simulink model "flyback_DT_working(2)"  (R2022b)
settings: Solver=FixedStepDiscrete  StartTime=0.0  StopTime=100e-3  RelTol=1e-3
undefined symbols (not defined in the file): DiscIntNeverNeededParam
libraries: cstblocks x4, simulink x1
Description:
  | Symmetric FIR Filter
  | This example shows how to use HDL Coder(TM) to check, generate,
  | and verify HDL for a fixed-point symmetric FIR filter.
settings Model: DataTypeOverride=Off  Creator=The MathWorks, Inc.  LastModifiedBy=justu
settings SolverCC: AlgebraicLoopSolver=TrustRegion  AutoInsertRateTranBlk=on
settings DataIOCC: LimitDataPoints=on  SaveFormat=Array  SaveOutput=off  SignalLogging=off  SaveTime=off  ReturnWorkspaceOutputs=off  SignalLoggingName=logsOut
settings OptimizationCC: BlockReduction=off  BooleanDataType=off  ConditionallyExecuteInputs=off  DefaultParameterBehavior=Inlined  InheritOutputTypeSmallerThanSingle=on  InlineInvariantSignals=on  ExpressionDepthLimit=2147483647  InitFltsAndDblsToZero=on  LifeSpan=inf  BufferReusableBoundary=off
settings DebuggingCC: AlgebraicLoopMsg=error  SaveWithParameterizedLinksMsg=none  UnderspecifiedInitializationDetection=Classic  MergeDetectMultiDrivingBlocksExec=none  CheckExecutionContextPreStartOutputMsg=on  SignalResolutionControl=TryResolveAllWithWarning  MultiTaskDSMMsg=warning  MultiTaskCondExecSysMsg=none  SingleTaskRateTransMsg=error  IntegerOverflowMsg=none  ParameterPrecisionLossMsg=none  FcnCallInpInsideContextMsg=warning  UnconnectedInputMsg=warning  UnconnectedOutputMsg=warning  UnconnectedLineMsg=warning  BusObjectLabelMismatch=none  StateNameClashWarn=warning  SFUnexpectedBacktrackingDiag=warning  SFNoUnconditionalDefaultTransitionDiag=warning  SFExecutionAtInitializationDiag=none  SFMachineParentedDataDiag=warning  IntegerSaturationMsg=none  ArithmeticOperatorsInVariantConditions=warning
settings HardwareCC: ProdBitPerPointer=32  ProdBitPerSizeT=32  ProdBitPerPtrDiffT=32  ProdLargestAtomicFloat=None  ProdIntDivRoundTo=Undefined  ProdEndianess=Unspecified  ProdWordSize=32  ProdHWDeviceType=ASIC/FPGA  TargetUnknown=on  ProdEqTarget=off
settings ModelReferenceCC: EnableRefExpFcnMdlSchedulingChecks=on  PropagateSignalLabelsOutOfModel=off
settings SFSimCC: SimUseLocalCustomCode=off  CustomCodeUndefinedFunction=UseInterfaceOnly
settings RTWCC: RTWUseLocalCustomCode=off  DLArmComputeVersion=19.05
settings CodeAppCC: StateflowObjectComments=on
settings GRTTargetCC: TargetFcnLib=ansi_tfl_tmw.mat  TargetLangStandard=C89/C90 (ANSI)  CombineOutputUpdateFcns=off  GRTInterface=on
settings ConfigComp: CovMetricSettings=dw  CovSaveCumulativeToWorkspaceVar=on  CovSaveSingleToWorkspaceVar=on  CovExternalEMLEnable=off

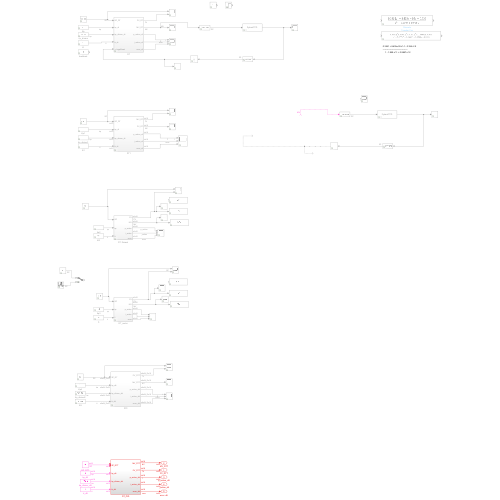
[thumbnail: Simulink's stored preview of the top-level diagram]
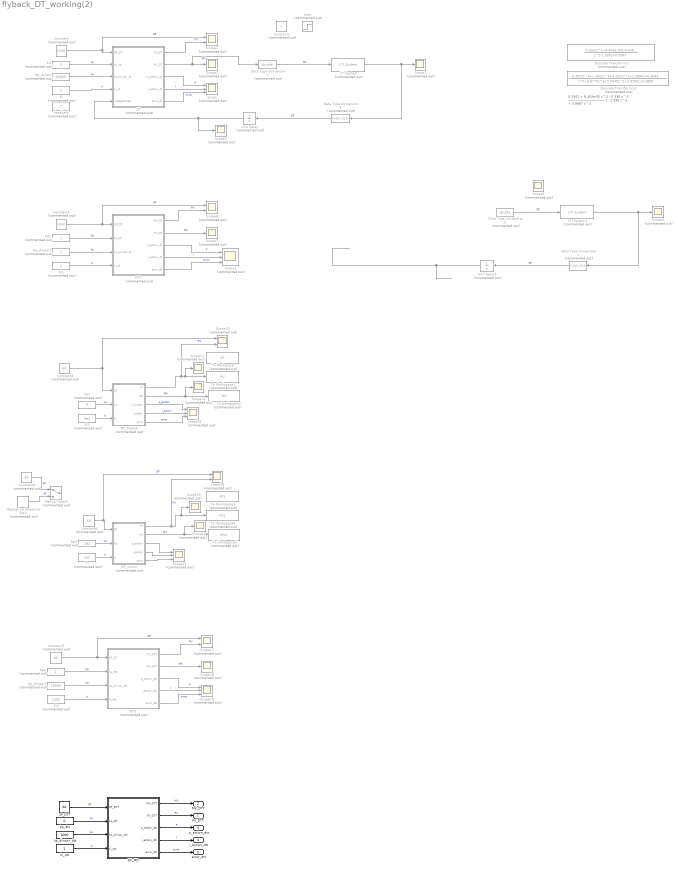
== system flyback_DT_working(2) ==
  note: 0.3361 + 8.403e-05 z^-1 - 0.336 z^-2
      |   ------------------------------------
      |       1 - 1.999 z^-1 + 0.9987 z^-2
  Constant : Constant  Commented=on  Value=10000  OutDataTypeStr=fixdt(1,16,0)
  Constant1 : Constant  Commented=on  OutDataTypeStr=fixdt(1,16,0)
  Constant2 : Constant  Commented=on  Value=10000  OutDataTypeStr=fixdt(1,16,0)
  Constant3 : Constant  Commented=on  Value=60  OutDataTypeStr=fixdt(1,64,32)
  Constant4 : Constant  Commented=on  Value=50  OutDataTypeStr=fixdt(1,16,0)
  Constant5 : Constant  Commented=on  Value=60  OutDataTypeStr=fixdt(1,64,32)
  Constant6 : Constant  Commented=on  Value=50  OutDataTypeStr=fixdt(1,16,0)
  DT : Subsystem  Commented=on
  DT1 : Subsystem  Commented=on
  DT2 : Subsystem  Commented=on
  DT_PID : Subsystem
  DT_flyback : Subsystem  Commented=on
  DT_motor : Subsystem  Commented=on
  Data Type Conversion1 : DataTypeConversion  Commented=on  OutDataTypeStr=double  SaturateOnIntegerOverflow=off  RndMeth=Floor
  Data Type Conversion2 : DataTypeConversion  Commented=on  OutDataTypeStr=double  SaturateOnIntegerOverflow=off  RndMeth=Floor
  Data Type Conversion3 : DataTypeConversion  Commented=on  OutDataTypeStr=fixdt(1,16,0)  SaturateOnIntegerOverflow=off  RndMeth=Floor
  Data Type Conversion5 : DataTypeConversion  Commented=on  OutDataTypeStr=fixdt(1,16,0)  SaturateOnIntegerOverflow=off  RndMeth=Floor
  Discrete Transfer Fcn : DiscreteTransferFcn  Commented=on  Numerator=[0.3361 8.403e-05 -0.336]  Denominator=[1 -1.999 0.9987]  SampleTime=1e-5  a0EqualsOne=on
  Discrete Transfer Fcn2 : DiscreteTransferFcn  Commented=on  Numerator=[0.3677 1.4652 2.1917 1.4584 0.3643]  Denominator=[1 3.9779 5.9449 3.9560 0.9890]  SampleTime=0.00001  NumCoefDataTypeStr=fixdt(1,64,32)  DenCoefDataTypeStr=fixdt(1,64,32)  NumProductDataTypeStr=fixdt(1,64,32)  DenProductDataTypeStr=fixdt(1,64,32)  NumAccumDataTypeStr=fixdt(1,64,32)  DenAccumDataTypeStr=fixdt(1,64,32)  OutDataTypeStr=fixdt(1,64,32)
  Ki : Constant  Commented=on  OutDataTypeStr=fixdt(1,16,0)
  Ki1 : Constant  Commented=on  OutDataTypeStr=fixdt(1,16,0)
  Ki2 : Constant  Commented=on  Value=5e3  OutDataTypeStr=fixdt(1,64,32)
  Ki3 : Constant  Commented=on  Value=1000  OutDataTypeStr=fixdt(1,64,32)
  Kp : Constant  Commented=on  Value=0  OutDataTypeStr=fixdt(1,16,0)
  Kp1 : Constant  Commented=on  OutDataTypeStr=fixdt(1,16,0)
  Kp2 : Constant  Commented=on  Value=0  OutDataTypeStr=fixdt(1,64,32)
  Kp3 : Constant  Commented=on  Value=1e2  OutDataTypeStr=fixdt(1,16,0)
  Kp4 : Constant  Commented=on  OutDataTypeStr=fixdt(1,64,32)
  Kp_divisor : Constant  Commented=on  Value=10000  OutDataTypeStr=fixdt(1,16,0)
  Kp_divisor1 : Constant  Commented=on  OutDataTypeStr=fixdt(1,16,0)
  Kp_divisor2 : Constant  Commented=on  Value=10000  OutDataTypeStr=fixdt(1,64,32)
  LTI System : cstblocks/LTI System  Commented=on  sys=flybackTFD  IC=[]
  LTI System1 : cstblocks/LTI System  Commented=on  sys=flybackTFD  IC=[]
  Manual Switch : ManualSwitch  Commented=on
  Repeating Sequence Stair : simulink/Sources/Repeating Sequence Stair  Commented=on  OutValues=[8 4 20 50 5 10].'  tsamp=0.1/6  OutMin=[]  OutMax=[]  OutDataTypeStr=double  OutputDataTypeScalingMode=double  OutDataType=fixdt(0,8)  ConRadixGroup=Best Precision: Vector-wise  OutScaling=2^-12
  SP_DTT : Constant  Value=60  OutDataTypeStr=fixdt(1,16,0)
  Scope{,5,10,13,16} (5 alike) : Scope  Commented=on  NumInputPorts=3
  Scope{1,6,17,19..20} (5 alike) : Scope  Commented=on  NumInputPorts=2
  Scope{2..4,7..9,11..12,14..15,18} (11 alike) : Scope  Commented=on
  Step : Step  Commented=on  Time=0  After=30  SampleTime=0
  Ti : Constant  Commented=on  Value=1e2  OutDataTypeStr=fixdt(1,16,0)
  To Workspace : ToWorkspace  Commented=on  VariableName=SP  SaveFormat=Structure With Time  SampleTime=-1
  To Workspace1 : ToWorkspace  Commented=on  VariableName=PV  SaveFormat=Structure With Time  SampleTime=-1
  To Workspace2 : ToWorkspace  Commented=on  VariableName=MV  SaveFormat=Structure With Time  SampleTime=-1
  To Workspace3 : ToWorkspace  Commented=on  VariableName=SP1  SaveFormat=Structure With Time  SampleTime=-1
  To Workspace4 : ToWorkspace  Commented=on  VariableName=PV1  SaveFormat=Structure With Time  SampleTime=-1
  To Workspace5 : ToWorkspace  Commented=on  VariableName=MV1  SaveFormat=Structure With Time  SampleTime=-1
  Unit Delay : UnitDelay  Commented=on  SampleTime=-1  HasFrameUpgradeWarning=on
  Unit Delay1 : UnitDelay  Commented=on  SampleTime=-1  HasFrameUpgradeWarning=on
  feedback : Constant  Commented=on  OutDataTypeStr=fixdt(1,16,0)
  ki_dtt : Constant  OutDataTypeStr=fixdt(1,16,0)
  kp_divisor_dtt : Constant  Value=1000  OutDataTypeStr=fixdt(1,16,0)
  kp_dtt : Constant  Value=0  OutDataTypeStr=fixdt(1,16,0)
  PV_DTT : Outport  OutDataTypeStr=fixdt(1,16,0)  SampleTime=0.00001  VectorParamsAs1DForOutWhenUnconnected=off
  MV_DTT : Outport  Port=2  OutDataTypeStr=fixdt(1,16,0)  SampleTime=0.00001  VectorParamsAs1DForOutWhenUnconnected=off
  p_action_dtt : Outport  Port=3  OutDataTypeStr=fixdt(1,16,0)  SampleTime=0.00001  VectorParamsAs1DForOutWhenUnconnected=off
  i_action_dtt : Outport  Port=4  OutDataTypeStr=fixdt(1,16,0)  SampleTime=0.00001  VectorParamsAs1DForOutWhenUnconnected=off
  error_dtt : Outport  Port=5  OutDataTypeStr=fixdt(1,16,0)  SampleTime=0.00001  VectorParamsAs1DForOutWhenUnconnected=off
  wires:
  Kp/1 -> DT/2(kp_dt)  "kp"
  Ki/1 -> DT/4(ki_dt)  "ti"
  Constant/1 -> DT/1(SP_DT), Scope1/1  "SP"
  DT/3(p_action_dt) -> Scope/1  "P"
  DT/5(error_dt) -> Scope/3  "error"
  DT/1(PV_DT) -> Scope1/2  "PV"
  DT/4(i_action_dt) -> Scope/2  "I"
  Kp_divisor/1 -> DT/3(kp_divisor_dt)  "kp"
  Data Type Conversion1/1 -> LTI System/1  "SP"
  Data Type Conversion5/1 -> Unit Delay/1  "SP"
  Unit Delay/1 -> DT/5(voltageRead), Scope4/1
  DT/2(MV_DT) -> Data Type Conversion1/1, Scope2/1  "MV"
  LTI System/1 -> Data Type Conversion5/1, Scope3/1
  DT1/2(PV_DT) -> Scope7/1  "MV"
  Kp_divisor1/1 -> DT1/3(kp_divisor_dt)  "kp"
  DT1/4(i_action_dt) -> Scope5/2  "I"
  DT1/1(MV_DT) -> Scope6/2  "PV"
  DT1/5(error_dt) -> Scope5/3  "error"
  DT1/3(p_action_dt) -> Scope5/1  "P"
  Constant2/1 -> Scope6/1, DT1/1(SP_DT)  "SP"
  Ki1/1 -> DT1/4(ki_dt)  "ti"
  Kp1/1 -> DT1/2(kp_dt)  "kp"
  Data Type Conversion3/1 -> Unit Delay1/1  "SP"
  LTI System1/1 -> Scope8/1, Data Type Conversion3/1
  Unit Delay1/1 -> ?
  Data Type Conversion2/1 -> LTI System1/1  "SP"
  ? -> Data Type Conversion2/1  "MV"
  DT_flyback/4(i_action) -> Scope10/2  "i_action"
  Kp2/1 -> DT_flyback/2(kp)  "kp"
  DT_flyback/1(PV) -> Scope20/2, Scope11/1, To Workspace1/1  "PV"
  DT_flyback/2(MV) -> Scope12/1, To Workspace2/1  "MV"
  DT_flyback/5(error) -> Scope10/3  "error"
  DT_flyback/3(p_action) -> Scope10/1  "p_action"
  Ki2/1 -> DT_flyback/3(ki)  "ti"
  DT_motor/1(PV) -> Scope19/2, Scope15/1, To Workspace4/1  "PV"
  DT_motor/2(MV) -> Scope14/1, To Workspace5/1  "MV"
  DT_motor/5(error) -> Scope13/3
  DT_motor/3(p_action) -> Scope13/1
  Ti/1 -> DT_motor/3(ti)  "ti"
  Kp3/1 -> DT_motor/2(kp)  "kp"
  DT_motor/4(i_action) -> Scope13/2
  DT2/2(MV_DTT) -> Scope18/1  "MV"
  DT2/4(i_action_dtt) -> Scope16/2  "I"
  Kp_divisor2/1 -> DT2/3(kp_divisor_dtt)  "kp"
  DT2/3(p_action_dtt) -> Scope16/1  "P"
  Ki3/1 -> DT2/4(ki_dtt)  "ti"
  DT2/5(error_dtt) -> Scope16/3  "error"
  DT2/1(PV_DTT) -> Scope17/2  "PV"
  Constant5/1 -> Scope17/1, DT2/1(SP_DT)  "SP"
  Kp4/1 -> DT2/2(kp_dtt)  "kp"
  Constant6/1 -> Scope19/1, DT_motor/1(SP)  "SP"
  Repeating Sequence Stair/1 -> Manual Switch/2  "SP"
  Constant4/1 -> Manual Switch/1  "SP"
  Constant3/1 -> Scope20/1, DT_flyback/1(SP)
  DT_PID/5(error_dtt) -> error_dtt/1  "error"
  DT_PID/2(PV_DTT) -> PV_DTT/1  "PV"
  DT_PID/4(i_action_dtt) -> i_action_dtt/1  "I"
  DT_PID/3(p_action_dtt) -> p_action_dtt/1  "P"
  DT_PID/1(MV_DTT) -> MV_DTT/1  "MV"
  kp_dtt/1 -> DT_PID/2(kp_dtt)  "kp"
  SP_DTT/1 -> DT_PID/1(SP_DTT)  "SP"
  kp_divisor_dtt/1 -> DT_PID/3(kp_divisor_dtt)  "kp"
  ki_dtt/1 -> DT_PID/4(ki_dtt)  "ti"

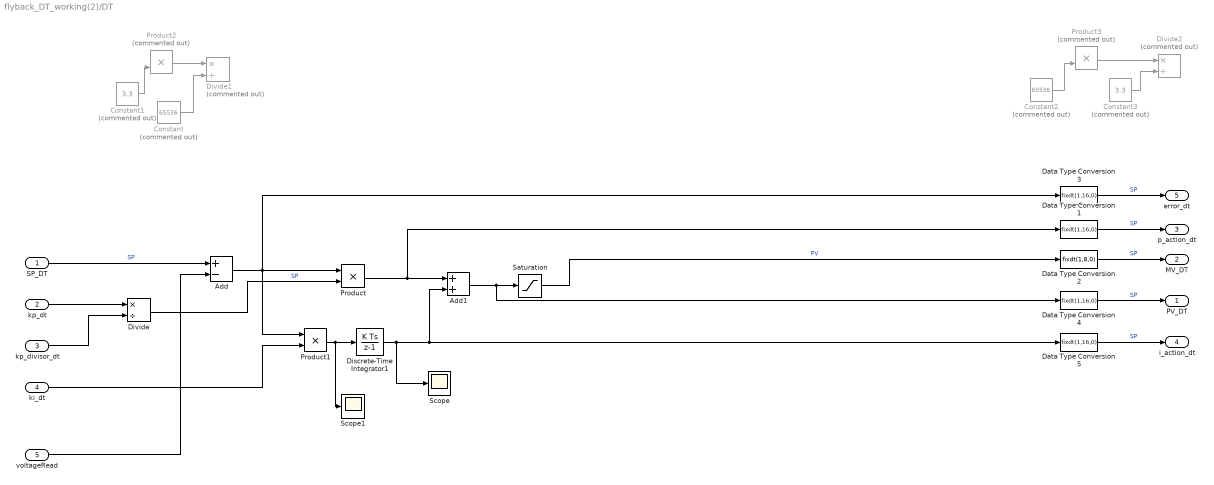
== system flyback_DT_working(2)/DT ==
  SP_DT : Inport  OutDataTypeStr=fixdt(1,16,0)  SampleTime=0.00001
  kp_dt : Inport  Port=2  OutDataTypeStr=fixdt(1,16,0)  SampleTime=0.00001
  kp_divisor_dt : Inport  Port=3  OutDataTypeStr=fixdt(1,16,0)  SampleTime=0.00001
  ki_dt : Inport  Port=4  OutDataTypeStr=fixdt(1,16,0)  SampleTime=0.00001
  voltageRead : Inport  Port=5  OutDataTypeStr=fixdt(1,16,0)
  Add : Sum  Inputs=+-  AccumDataTypeStr=fixdt(1,64,32)  OutDataTypeStr=fixdt(1,64,32)
  Add1 : Sum  AccumDataTypeStr=fixdt(1,64,32)  OutDataTypeStr=fixdt(1,64,32)
  Constant : Constant  Commented=on  Value=65536  OutDataTypeStr=fixdt(1,64,32)
  Constant1 : Constant  Commented=on  Value=3.3  OutDataTypeStr=fixdt(1,64,32)
  Constant2 : Constant  Commented=on  Value=65536  OutDataTypeStr=fixdt(1,64,32)
  Constant3 : Constant  Commented=on  Value=3.3  OutDataTypeStr=fixdt(1,64,32)
  Data Type Conversion{1,3..5} (4 alike) : DataTypeConversion  OutDataTypeStr=fixdt(1,16,0)  SaturateOnIntegerOverflow=off  RndMeth=Floor
  Data Type Conversion2 : DataTypeConversion  OutDataTypeStr=fixdt(1,8,0)  SaturateOnIntegerOverflow=off  RndMeth=Floor
  Discrete-Time Integrator1 : DiscreteIntegrator  SampleTime=0.00001  OutDataTypeStr=fixdt(1,64,32)  ICPrevOutput=DiscIntNeverNeededParam  ICPrevScaledInput=DiscIntNeverNeededParam
  Divide : Product  Inputs=*/  RndMeth=Zero  SaturateOnIntegerOverflow=on  LockScale=on
  Divide1 : Product  Commented=on  Inputs=*/  RndMeth=Zero  SaturateOnIntegerOverflow=on  LockScale=on
  Divide2 : Product  Commented=on  Inputs=*/  RndMeth=Zero  SaturateOnIntegerOverflow=on  LockScale=on
  Product : Product  OutDataTypeStr=fixdt(1,64,32)
  Product1 : Product  OutDataTypeStr=fixdt(1,64,32)
  Product2 : Product  Commented=on  OutDataTypeStr=fixdt(1,64,32)
  Product3 : Product  Commented=on  OutDataTypeStr=fixdt(1,64,32)
  Saturation : Saturate  UpperLimit=255  LowerLimit=0  OutDataTypeStr=fixdt(1,64,32)
  Scope : Scope
  Scope1 : Scope
  PV_DT : Outport  OutDataTypeStr=fixdt(1,16,0)  SampleTime=0.00001  VectorParamsAs1DForOutWhenUnconnected=off
  MV_DT : Outport  Port=2  OutDataTypeStr=fixdt(1,8,0)  SampleTime=0.00001  VectorParamsAs1DForOutWhenUnconnected=off
  p_action_dt : Outport  Port=3  OutDataTypeStr=fixdt(1,16,0)  SampleTime=0.00001  VectorParamsAs1DForOutWhenUnconnected=off
  i_action_dt : Outport  Port=4  OutDataTypeStr=fixdt(1,16,0)  SampleTime=0.00001  VectorParamsAs1DForOutWhenUnconnected=off
  error_dt : Outport  Port=5  OutDataTypeStr=fixdt(1,16,0)  SampleTime=0.00001  VectorParamsAs1DForOutWhenUnconnected=off
  wires:
  Product1/1 -> Scope1/1, Discrete-Time Integrator1/1
  Add/1 -> Data Type Conversion3/1, Product/1, Product1/1
  Product/1 -> Data Type Conversion1/1, Add1/1
  Saturation/1 -> Data Type Conversion2/1  "PV"
  Discrete-Time Integrator1/1 -> Scope/1, Data Type Conversion5/1, Add1/2
  Data Type Conversion1/1 -> p_action_dt/1  "SP"
  Data Type Conversion3/1 -> error_dt/1  "SP"
  Data Type Conversion2/1 -> MV_DT/1  "SP"
  Data Type Conversion4/1 -> PV_DT/1  "SP"
  Data Type Conversion5/1 -> i_action_dt/1  "SP"
  ki_dt/1 -> Product1/2
  kp_dt/1 -> Divide/1
  kp_divisor_dt/1 -> Divide/2
  Divide/1 -> Product/2  "SP"
  Add1/1 -> Data Type Conversion4/1, Saturation/1
  SP_DT/1 -> Add/1  "SP"
  Product2/1 -> Divide1/1
  Constant1/1 -> Product2/2
  Constant/1 -> Divide1/2
  Constant3/1 -> Divide2/2
  Constant2/1 -> Product3/2
  Product3/1 -> Divide2/1
  voltageRead/1 -> Add/2

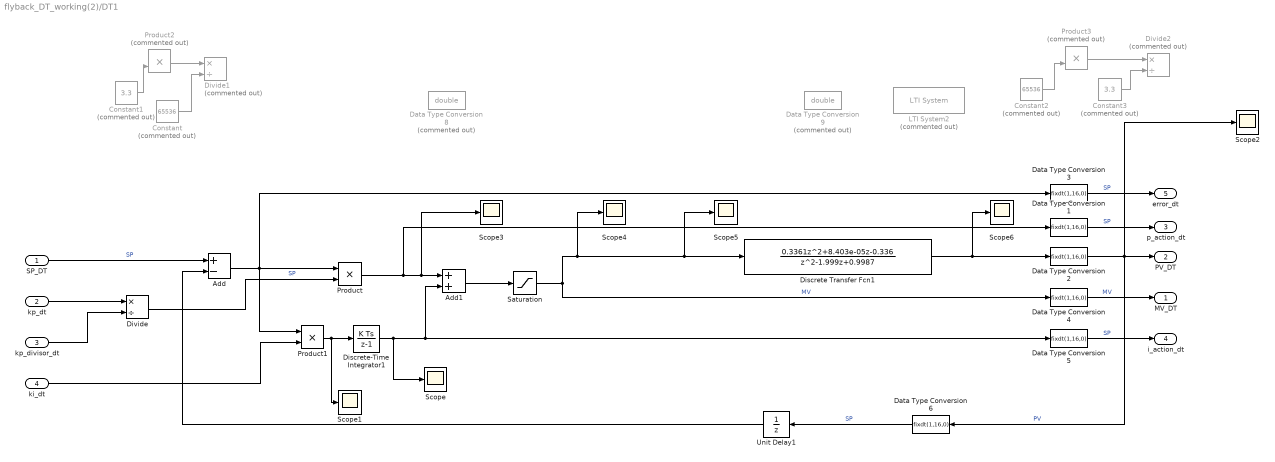
== system flyback_DT_working(2)/DT1 ==
  SP_DT : Inport  OutDataTypeStr=fixdt(1,16,0)  SampleTime=0.00001
  kp_dt : Inport  Port=2  OutDataTypeStr=fixdt(1,16,0)  SampleTime=0.00001
  kp_divisor_dt : Inport  Port=3  OutDataTypeStr=fixdt(1,16,0)  SampleTime=0.00001
  ki_dt : Inport  Port=4  OutDataTypeStr=fixdt(1,16,0)  SampleTime=0.00001
  Add : Sum  Inputs=+-  AccumDataTypeStr=fixdt(1,64,32)  OutDataTypeStr=fixdt(1,64,32)
  Add1 : Sum  AccumDataTypeStr=fixdt(1,64,32)  OutDataTypeStr=fixdt(1,64,32)
  Constant : Constant  Commented=on  Value=65536  OutDataTypeStr=fixdt(1,64,32)
  Constant1 : Constant  Commented=on  Value=3.3  OutDataTypeStr=fixdt(1,64,32)
  Constant2 : Constant  Commented=on  Value=65536  OutDataTypeStr=fixdt(1,64,32)
  Constant3 : Constant  Commented=on  Value=3.3  OutDataTypeStr=fixdt(1,64,32)
  Data Type Conversion{1..6} (6 alike) : DataTypeConversion  OutDataTypeStr=fixdt(1,16,0)  SaturateOnIntegerOverflow=off  RndMeth=Floor
  Data Type Conversion8 : DataTypeConversion  Commented=on  OutDataTypeStr=double  SaturateOnIntegerOverflow=off  RndMeth=Floor
  Data Type Conversion9 : DataTypeConversion  Commented=on  OutDataTypeStr=double  SaturateOnIntegerOverflow=off  RndMeth=Floor
  Discrete Transfer Fcn1 : DiscreteTransferFcn  Numerator=[0.3361 8.403e-05 -0.336]  Denominator=[1 -1.999 0.9987]  SampleTime=1e-5  a0EqualsOne=on
  Discrete-Time Integrator1 : DiscreteIntegrator  SampleTime=0.00001  OutDataTypeStr=fixdt(1,64,32)  ICPrevOutput=DiscIntNeverNeededParam  ICPrevScaledInput=DiscIntNeverNeededParam
  Divide : Product  Inputs=*/  RndMeth=Zero  SaturateOnIntegerOverflow=on  LockScale=on
  Divide1 : Product  Commented=on  Inputs=*/  RndMeth=Zero  SaturateOnIntegerOverflow=on  LockScale=on
  Divide2 : Product  Commented=on  Inputs=*/  RndMeth=Zero  SaturateOnIntegerOverflow=on  LockScale=on
  LTI System2 : cstblocks/LTI System  Commented=on  sys=flybackTFD  IC=[]
  Product : Product  OutDataTypeStr=fixdt(1,64,32)
  Product1 : Product  OutDataTypeStr=fixdt(1,64,32)
  Product2 : Product  Commented=on  OutDataTypeStr=fixdt(1,64,32)
  Product3 : Product  Commented=on  OutDataTypeStr=fixdt(1,64,32)
  Saturation : Saturate  UpperLimit=255  LowerLimit=0  OutDataTypeStr=fixdt(1,64,32)
  Scope{,1..6} (7 alike) : Scope
  Unit Delay1 : UnitDelay  SampleTime=1e-5  HasFrameUpgradeWarning=on
  MV_DT : Outport  OutDataTypeStr=fixdt(1,16,0)  SampleTime=0.00001  VectorParamsAs1DForOutWhenUnconnected=off
  PV_DT : Outport  Port=2  OutDataTypeStr=fixdt(1,16,0)  SampleTime=0.00001  VectorParamsAs1DForOutWhenUnconnected=off
  p_action_dt : Outport  Port=3  OutDataTypeStr=fixdt(1,16,0)  SampleTime=0.00001  VectorParamsAs1DForOutWhenUnconnected=off
  i_action_dt : Outport  Port=4  OutDataTypeStr=fixdt(1,16,0)  SampleTime=0.00001  VectorParamsAs1DForOutWhenUnconnected=off
  error_dt : Outport  Port=5  OutDataTypeStr=fixdt(1,16,0)  SampleTime=0.00001  VectorParamsAs1DForOutWhenUnconnected=off
  wires:
  Product3/1 -> Divide2/1
  Constant2/1 -> Product3/2
  Constant3/1 -> Divide2/2
  Constant/1 -> Divide1/2
  Constant1/1 -> Product2/2
  Product2/1 -> Divide1/1
  SP_DT/1 -> Add/1  "SP"
  Add1/1 -> Saturation/1
  Divide/1 -> Product/2  "SP"
  kp_divisor_dt/1 -> Divide/2
  kp_dt/1 -> Divide/1
  ki_dt/1 -> Product1/2
  Data Type Conversion5/1 -> i_action_dt/1  "SP"
  Data Type Conversion4/1 -> MV_DT/1  "MV"
  Data Type Conversion2/1 -> Data Type Conversion6/1, Scope2/1, PV_DT/1  "PV"
  Data Type Conversion3/1 -> error_dt/1  "SP"
  Data Type Conversion1/1 -> p_action_dt/1  "SP"
  Discrete-Time Integrator1/1 -> Add1/2, Data Type Conversion5/1, Scope/1
  Product/1 -> Scope3/1, Add1/1, Data Type Conversion1/1
  Add/1 -> Product1/1, Product/1, Data Type Conversion3/1
  Product1/1 -> Discrete-Time Integrator1/1, Scope1/1
  Discrete Transfer Fcn1/1 -> Scope6/1, Data Type Conversion2/1
  Data Type Conversion6/1 -> Unit Delay1/1  "SP"
  Unit Delay1/1 -> Add/2
  Saturation/1 -> Data Type Conversion4/1, Scope5/1, Discrete Transfer Fcn1/1, Scope4/1  "MV"

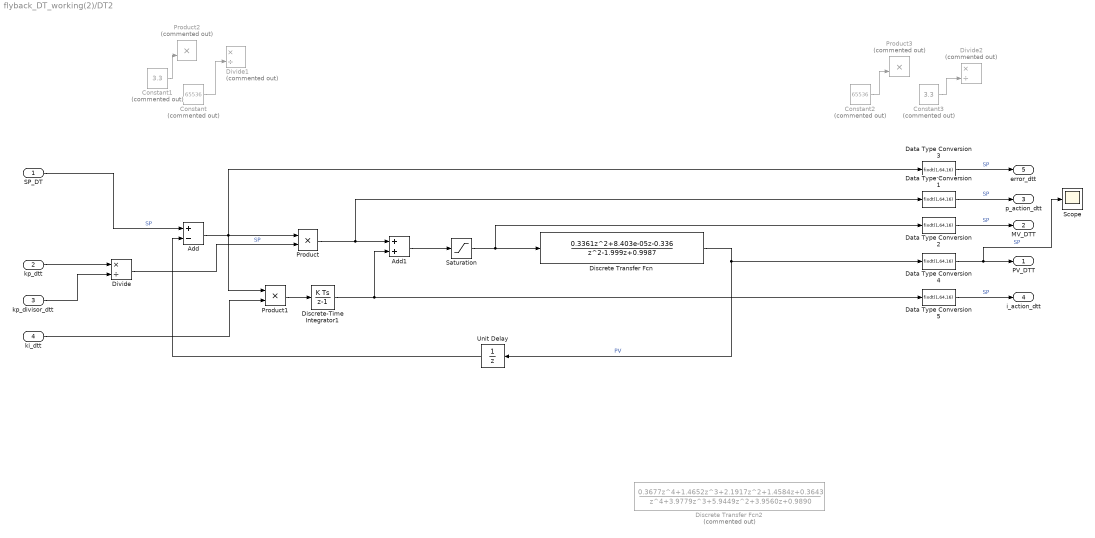
== system flyback_DT_working(2)/DT2 ==
  SP_DT : Inport  OutDataTypeStr=fixdt(1,64,32)  SampleTime=0.00001
  kp_dtt : Inport  Port=2  OutDataTypeStr=fixdt(1,64,32)  SampleTime=0.00001
  kp_divisor_dtt : Inport  Port=3  OutDataTypeStr=fixdt(1,64,32)  SampleTime=0.00001
  ki_dtt : Inport  Port=4  OutDataTypeStr=fixdt(1,64,32)  SampleTime=0.00001
  Add : Sum  Inputs=+-  AccumDataTypeStr=fixdt(1,64,32)  OutDataTypeStr=fixdt(1,64,32)
  Add1 : Sum  AccumDataTypeStr=fixdt(1,64,32)  OutDataTypeStr=fixdt(1,64,32)
  Constant : Constant  Commented=on  Value=65536  OutDataTypeStr=fixdt(1,64,32)
  Constant1 : Constant  Commented=on  Value=3.3  OutDataTypeStr=fixdt(1,64,32)
  Constant2 : Constant  Commented=on  Value=65536  OutDataTypeStr=fixdt(1,64,32)
  Constant3 : Constant  Commented=on  Value=3.3  OutDataTypeStr=fixdt(1,64,32)
  Data Type Conversion{1..5} (5 alike) : DataTypeConversion  OutDataTypeStr=fixdt(1,64,16)  SaturateOnIntegerOverflow=off  RndMeth=Floor
  Discrete Transfer Fcn : DiscreteTransferFcn  Numerator=[0.3361 8.403e-05 -0.336]  Denominator=[1 -1.999 0.9987]  SampleTime=1e-5  a0EqualsOne=on
  Discrete Transfer Fcn2 : DiscreteTransferFcn  Commented=on  Numerator=[0.3677 1.4652 2.1917 1.4584 0.3643]  Denominator=[1 3.9779 5.9449 3.9560 0.9890]  SampleTime=0.00001  NumCoefDataTypeStr=fixdt(1,64,32)  DenCoefDataTypeStr=fixdt(1,64,32)  NumProductDataTypeStr=fixdt(1,64,32)  DenProductDataTypeStr=fixdt(1,64,32)  NumAccumDataTypeStr=fixdt(1,64,32)  DenAccumDataTypeStr=fixdt(1,64,32)  OutDataTypeStr=fixdt(1,64,32)
  Discrete-Time Integrator1 : DiscreteIntegrator  SampleTime=0.00001  OutDataTypeStr=fixdt(1,64,32)  ICPrevOutput=DiscIntNeverNeededParam  ICPrevScaledInput=DiscIntNeverNeededParam
  Divide : Product  Inputs=*/  RndMeth=Zero  SaturateOnIntegerOverflow=on  LockScale=on
  Divide1 : Product  Commented=on  Inputs=*/  RndMeth=Zero  SaturateOnIntegerOverflow=on  LockScale=on
  Divide2 : Product  Commented=on  Inputs=*/  RndMeth=Zero  SaturateOnIntegerOverflow=on  LockScale=on
  Product : Product  OutDataTypeStr=fixdt(1,64,32)
  Product1 : Product  OutDataTypeStr=fixdt(1,64,32)
  Product2 : Product  Commented=on  OutDataTypeStr=fixdt(1,64,32)
  Product3 : Product  Commented=on  OutDataTypeStr=fixdt(1,64,32)
  Saturation : Saturate  UpperLimit=255  LowerLimit=0  OutDataTypeStr=fixdt(1,64,32)
  Scope : Scope
  Unit Delay : UnitDelay  SampleTime=0.00001  HasFrameUpgradeWarning=on
  PV_DTT : Outport  OutDataTypeStr=fixdt(1,64,16)  SampleTime=0.00001  VectorParamsAs1DForOutWhenUnconnected=off
  MV_DTT : Outport  Port=2  OutDataTypeStr=fixdt(1,64,16)  SampleTime=0.00001  VectorParamsAs1DForOutWhenUnconnected=off
  p_action_dtt : Outport  Port=3  OutDataTypeStr=fixdt(1,64,16)  SampleTime=0.00001  VectorParamsAs1DForOutWhenUnconnected=off
  i_action_dtt : Outport  Port=4  OutDataTypeStr=fixdt(1,64,16)  SampleTime=0.00001  VectorParamsAs1DForOutWhenUnconnected=off
  error_dtt : Outport  Port=5  OutDataTypeStr=fixdt(1,64,16)  SampleTime=0.00001  VectorParamsAs1DForOutWhenUnconnected=off
  wires:
  Unit Delay/1 -> Add/2
  Product1/1 -> Discrete-Time Integrator1/1
  Add/1 -> Data Type Conversion3/1, Product/1, Product1/1
  Product/1 -> Data Type Conversion1/1, Add1/1
  Discrete Transfer Fcn/1 -> Data Type Conversion4/1, Unit Delay/1  "PV"
  Discrete-Time Integrator1/1 -> Data Type Conversion5/1, Add1/2
  Data Type Conversion1/1 -> p_action_dtt/1  "SP"
  Data Type Conversion3/1 -> error_dtt/1  "SP"
  Data Type Conversion2/1 -> MV_DTT/1  "SP"
  Data Type Conversion4/1 -> Scope/1, PV_DTT/1  "SP"
  Data Type Conversion5/1 -> i_action_dtt/1  "SP"
  ki_dtt/1 -> Product1/2
  kp_dtt/1 -> Divide/1
  kp_divisor_dtt/1 -> Divide/2
  Divide/1 -> Product/2  "SP"
  Add1/1 -> Saturation/1
  Saturation/1 -> Discrete Transfer Fcn/1, Data Type Conversion2/1
  SP_DT/1 -> Add/1  "SP"
  Constant2/1 -> Product3/2
  Constant3/1 -> Divide2/2
  Constant1/1 -> Product2/2
  Constant/1 -> Divide1/2

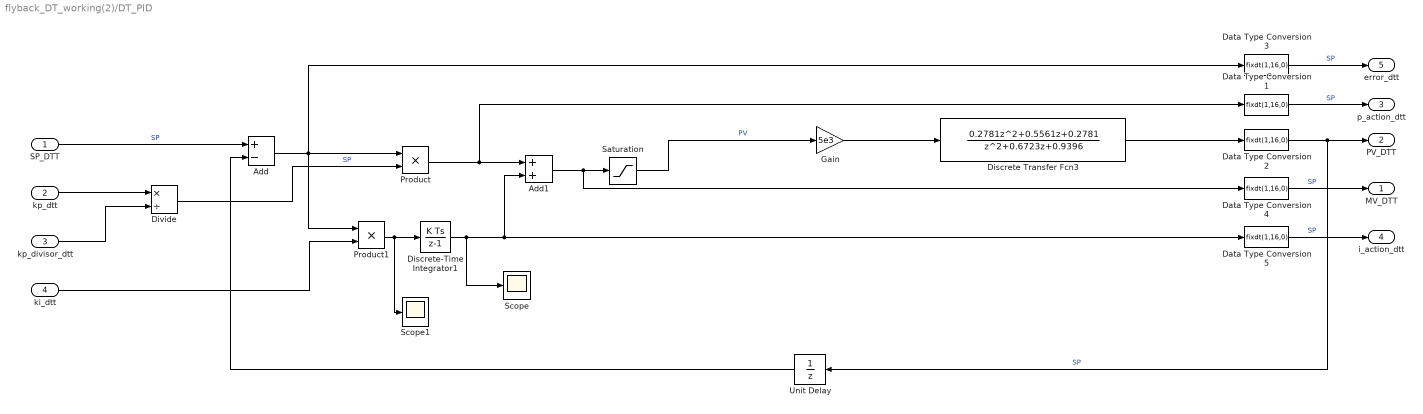
== system flyback_DT_working(2)/DT_PID ==
  SP_DTT : Inport  OutDataTypeStr=fixdt(1,16,0)  SampleTime=0.00001
  kp_dtt : Inport  Port=2  OutDataTypeStr=fixdt(1,16,0)  SampleTime=0.00001
  kp_divisor_dtt : Inport  Port=3  OutDataTypeStr=fixdt(1,16,0)  SampleTime=0.00001
  ki_dtt : Inport  Port=4  OutDataTypeStr=fixdt(1,16,0)  SampleTime=0.00001
  Add : Sum  Inputs=+-  AccumDataTypeStr=fixdt(1,64,32)  OutDataTypeStr=fixdt(1,64,32)
  Add1 : Sum  AccumDataTypeStr=fixdt(1,64,32)  OutDataTypeStr=fixdt(1,64,32)
  Data Type Conversion{1..5} (5 alike) : DataTypeConversion  OutDataTypeStr=fixdt(1,16,0)  SaturateOnIntegerOverflow=off  RndMeth=Floor
  Discrete Transfer Fcn3 : DiscreteTransferFcn  Numerator=[0.2781 0.5561 0.2781]  Denominator=[1 0.6723 0.9396]  SampleTime=1e-5  a0EqualsOne=on  NumCoefDataTypeStr=fixdt(1,64,32)  DenCoefDataTypeStr=fixdt(1,64,32)  NumProductDataTypeStr=fixdt(1,64,32)  DenProductDataTypeStr=fixdt(1,64,32)  NumAccumDataTypeStr=fixdt(1,64,32)  DenAccumDataTypeStr=fixdt(1,64,32)  OutDataTypeStr=fixdt(1,64,32)
  Discrete-Time Integrator1 : DiscreteIntegrator  SampleTime=0.00001  OutDataTypeStr=fixdt(1,64,32)  ICPrevOutput=DiscIntNeverNeededParam  ICPrevScaledInput=DiscIntNeverNeededParam
  Divide : Product  Inputs=*/  RndMeth=Zero  SaturateOnIntegerOverflow=on  LockScale=on
  Gain : Gain  Gain=5e3
  Product : Product  OutDataTypeStr=fixdt(1,64,32)
  Product1 : Product  OutDataTypeStr=fixdt(1,64,32)
  Saturation : Saturate  UpperLimit=255  LowerLimit=0  OutDataTypeStr=fixdt(1,64,32)
  Scope : Scope
  Scope1 : Scope
  Unit Delay : UnitDelay  SampleTime=-1  HasFrameUpgradeWarning=on
  MV_DTT : Outport  OutDataTypeStr=fixdt(1,16,0)  SampleTime=0.00001  VectorParamsAs1DForOutWhenUnconnected=off
  PV_DTT : Outport  Port=2  OutDataTypeStr=fixdt(1,16,0)  SampleTime=0.00001  VectorParamsAs1DForOutWhenUnconnected=off
  p_action_dtt : Outport  Port=3  OutDataTypeStr=fixdt(1,16,0)  SampleTime=0.00001  VectorParamsAs1DForOutWhenUnconnected=off
  i_action_dtt : Outport  Port=4  OutDataTypeStr=fixdt(1,16,0)  SampleTime=0.00001  VectorParamsAs1DForOutWhenUnconnected=off
  error_dtt : Outport  Port=5  OutDataTypeStr=fixdt(1,16,0)  SampleTime=0.00001  VectorParamsAs1DForOutWhenUnconnected=off
  wires:
  SP_DTT/1 -> Add/1  "SP"
  Add1/1 -> Saturation/1, Data Type Conversion4/1
  Divide/1 -> Product/2  "SP"
  kp_divisor_dtt/1 -> Divide/2
  kp_dtt/1 -> Divide/1
  ki_dtt/1 -> Product1/2
  Data Type Conversion5/1 -> i_action_dtt/1  "SP"
  Data Type Conversion4/1 -> MV_DTT/1  "SP"
  Data Type Conversion2/1 -> Unit Delay/1, PV_DTT/1  "SP"
  Data Type Conversion3/1 -> error_dtt/1  "SP"
  Data Type Conversion1/1 -> p_action_dtt/1  "SP"
  Discrete-Time Integrator1/1 -> Add1/2, Data Type Conversion5/1, Scope/1
  Saturation/1 -> Gain/1  "PV"
  Product/1 -> Add1/1, Data Type Conversion1/1
  Add/1 -> Product1/1, Product/1, Data Type Conversion3/1
  Product1/1 -> Discrete-Time Integrator1/1, Scope1/1
  Discrete Transfer Fcn3/1 -> Data Type Conversion2/1
  Unit Delay/1 -> Add/2
  Gain/1 -> Discrete Transfer Fcn3/1

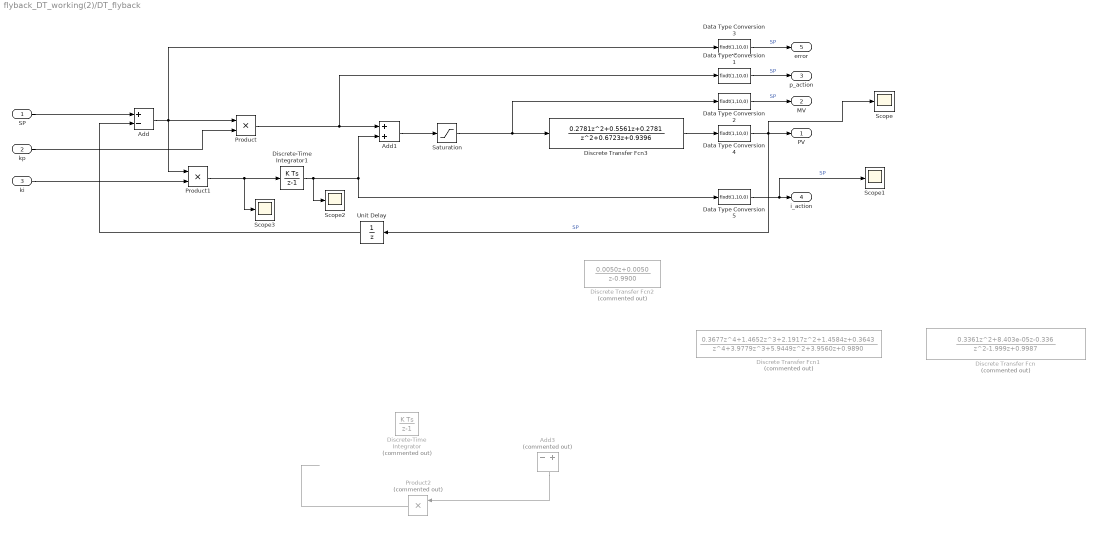
== system flyback_DT_working(2)/DT_flyback ==
  SP : Inport
  kp : Inport  Port=2
  ki : Inport  Port=3
  Add : Sum  Inputs=+-  AccumDataTypeStr=fixdt(1,64,32)  OutDataTypeStr=fixdt(1,64,32)
  Add1 : Sum  AccumDataTypeStr=fixdt(1,64,32)  OutDataTypeStr=fixdt(1,64,32)
  Add3 : Sum  Commented=on  Inputs=-+  AccumDataTypeStr=fixdt(1,64,32)  OutDataTypeStr=fixdt(1,64,32)
  Data Type Conversion{1..5} (5 alike) : DataTypeConversion  OutDataTypeStr=fixdt(1,10,0)  SaturateOnIntegerOverflow=off  RndMeth=Floor
  Discrete Transfer Fcn : DiscreteTransferFcn  Commented=on  Numerator=[0.3361 8.403e-05 -0.336]  Denominator=[1 -1.999 0.9987]  SampleTime=1e-5  a0EqualsOne=on  NumCoefDataTypeStr=fixdt(1,64,32)  DenCoefDataTypeStr=fixdt(1,64,32)  NumProductDataTypeStr=fixdt(1,64,32)  DenProductDataTypeStr=fixdt(1,64,32)  NumAccumDataTypeStr=fixdt(1,64,32)  DenAccumDataTypeStr=fixdt(1,64,32)  OutDataTypeStr=fixdt(1,64,32)
  Discrete Transfer Fcn1 : DiscreteTransferFcn  Commented=on  Numerator=[0.3677 1.4652 2.1917 1.4584 0.3643]  Denominator=[1 3.9779 5.9449 3.9560 0.9890]  SampleTime=0.00001  NumCoefDataTypeStr=fixdt(1,64,32)  DenCoefDataTypeStr=fixdt(1,64,32)  NumProductDataTypeStr=fixdt(1,64,32)  DenProductDataTypeStr=fixdt(1,64,32)  NumAccumDataTypeStr=fixdt(1,64,32)  DenAccumDataTypeStr=fixdt(1,64,32)  OutDataTypeStr=fixdt(1,64,32)
  Discrete Transfer Fcn2 : DiscreteTransferFcn  Commented=on  Numerator=[0.0050 0.0050]  Denominator=[1 -0.9900]  SampleTime=0.0001  NumCoefDataTypeStr=fixdt(1,64,32)  DenCoefDataTypeStr=fixdt(1,64,32)  NumProductDataTypeStr=fixdt(1,64,32)  DenProductDataTypeStr=fixdt(1,64,32)  NumAccumDataTypeStr=fixdt(1,64,32)  DenAccumDataTypeStr=fixdt(1,64,32)  OutDataTypeStr=fixdt(1,64,32)
  Discrete Transfer Fcn3 : DiscreteTransferFcn  Numerator=[0.2781 0.5561 0.2781]  Denominator=[1 0.6723 0.9396]  SampleTime=1e-5  a0EqualsOne=on  NumCoefDataTypeStr=fixdt(1,64,32)  DenCoefDataTypeStr=fixdt(1,64,32)  NumProductDataTypeStr=fixdt(1,64,32)  DenProductDataTypeStr=fixdt(1,64,32)  NumAccumDataTypeStr=fixdt(1,64,32)  DenAccumDataTypeStr=fixdt(1,64,32)  OutDataTypeStr=fixdt(1,64,32)
  Discrete-Time Integrator : DiscreteIntegrator  Commented=on  SampleTime=0.0001  OutDataTypeStr=fixdt(1,64,32)  ICPrevOutput=DiscIntNeverNeededParam  ICPrevScaledInput=DiscIntNeverNeededParam
  Discrete-Time Integrator1 : DiscreteIntegrator  SampleTime=0.00001  OutDataTypeStr=fixdt(1,64,32)  ICPrevOutput=DiscIntNeverNeededParam  ICPrevScaledInput=DiscIntNeverNeededParam
  Product : Product  OutDataTypeStr=fixdt(1,64,32)
  Product1 : Product  OutDataTypeStr=fixdt(1,64,32)
  Product2 : Product  Commented=on  OutDataTypeStr=fixdt(1,64,32)
  Saturation : Saturate  UpperLimit=255  LowerLimit=0  OutDataTypeStr=fixdt(1,64,32)
  Scope{,1..3} (4 alike) : Scope
  Unit Delay : UnitDelay  SampleTime=-1  HasFrameUpgradeWarning=on
  PV : Outport  OutDataTypeStr=fixdt(1,10,0)  SampleTime=0.001  VectorParamsAs1DForOutWhenUnconnected=off
  MV : Outport  Port=2  OutDataTypeStr=fixdt(1,10,0)  SampleTime=0.001  VectorParamsAs1DForOutWhenUnconnected=off
  p_action : Outport  Port=3  OutDataTypeStr=fixdt(1,10,0)  SampleTime=0.001  VectorParamsAs1DForOutWhenUnconnected=off
  i_action : Outport  Port=4  OutDataTypeStr=fixdt(1,10,0)  SampleTime=0.001  VectorParamsAs1DForOutWhenUnconnected=off
  error : Outport  Port=5  OutDataTypeStr=fixdt(1,10,0)  SampleTime=0.001  VectorParamsAs1DForOutWhenUnconnected=off
  wires:
  SP/1 -> Add/1
  Discrete Transfer Fcn3/1 -> Data Type Conversion4/1
  Add/1 -> Data Type Conversion3/1, Product/1, Product1/1
  kp/1 -> Product/2
  Product/1 -> Data Type Conversion1/1, Add1/1
  Discrete-Time Integrator1/1 -> Scope2/1, Add1/2, Data Type Conversion5/1
  Saturation/1 -> Discrete Transfer Fcn3/1, Data Type Conversion2/1
  Unit Delay/1 -> Add/2
  Add1/1 -> Saturation/1
  Data Type Conversion3/1 -> error/1  "SP"
  Data Type Conversion1/1 -> p_action/1  "SP"
  Data Type Conversion4/1 -> Unit Delay/1, Scope/1, PV/1  "SP"
  Data Type Conversion2/1 -> MV/1  "SP"
  Data Type Conversion5/1 -> Scope1/1, i_action/1  "SP"
  ? -> Add3/2
  Add3/1 -> Product2/1
  Product2/1 -> ?
  ? -> Add3/1
  ? -> Product2/2
  ki/1 -> Product1/2
  Product1/1 -> Scope3/1, Discrete-Time Integrator1/1

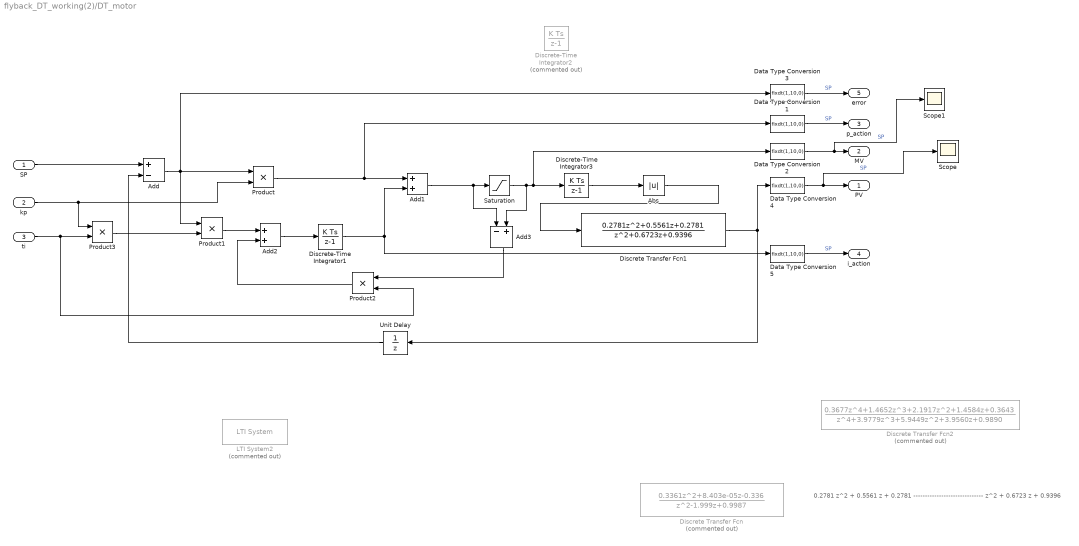
== system flyback_DT_working(2)/DT_motor ==
  note: 0.2781 z^2 + 0.5561 z + 0.2781 ------------------------------ z^2 + 0.6723 z + 0.9396
  SP : Inport
  kp : Inport  Port=2
  ti : Inport  Port=3
  Abs : Abs  SaturateOnIntegerOverflow=off
  Add : Sum  Inputs=+-  AccumDataTypeStr=fixdt(1,64,32)  OutDataTypeStr=fixdt(1,64,32)
  Add1 : Sum  AccumDataTypeStr=fixdt(1,64,32)  OutDataTypeStr=fixdt(1,64,32)
  Add2 : Sum  AccumDataTypeStr=fixdt(1,64,32)  OutDataTypeStr=fixdt(1,64,32)
  Add3 : Sum  Inputs=-+  AccumDataTypeStr=fixdt(1,64,32)  OutDataTypeStr=fixdt(1,64,32)
  Data Type Conversion{1..5} (5 alike) : DataTypeConversion  OutDataTypeStr=fixdt(1,10,0)  SaturateOnIntegerOverflow=off  RndMeth=Floor
  Discrete Transfer Fcn : DiscreteTransferFcn  Commented=on  Numerator=[0.3361 8.403e-05 -0.336]  Denominator=[1 -1.999 0.9987]  SampleTime=1e-5  a0EqualsOne=on  NumCoefDataTypeStr=fixdt(1,64,32)  DenCoefDataTypeStr=fixdt(1,64,32)  NumProductDataTypeStr=fixdt(1,64,32)  DenProductDataTypeStr=fixdt(1,64,32)  NumAccumDataTypeStr=fixdt(1,64,32)  DenAccumDataTypeStr=fixdt(1,64,32)  OutDataTypeStr=fixdt(1,64,32)
  Discrete Transfer Fcn1 : DiscreteTransferFcn  Numerator=[0.2781 0.5561 0.2781]  Denominator=[1 0.6723 0.9396]  SampleTime=1e-5  a0EqualsOne=on  NumCoefDataTypeStr=fixdt(1,64,32)  DenCoefDataTypeStr=fixdt(1,64,32)  NumProductDataTypeStr=fixdt(1,64,32)  DenProductDataTypeStr=fixdt(1,64,32)  NumAccumDataTypeStr=fixdt(1,64,32)  DenAccumDataTypeStr=fixdt(1,64,32)  OutDataTypeStr=fixdt(1,64,32)
  Discrete Transfer Fcn2 : DiscreteTransferFcn  Commented=on  Numerator=[0.3677 1.4652 2.1917 1.4584 0.3643]  Denominator=[1 3.9779 5.9449 3.9560 0.9890]  SampleTime=1e-5  NumCoefDataTypeStr=fixdt(1,64,32)  DenCoefDataTypeStr=fixdt(1,64,32)  NumProductDataTypeStr=fixdt(1,64,32)  DenProductDataTypeStr=fixdt(1,64,32)  NumAccumDataTypeStr=fixdt(1,64,32)  DenAccumDataTypeStr=fixdt(1,64,32)  OutDataTypeStr=fixdt(1,64,32)
  Discrete-Time Integrator1 : DiscreteIntegrator  SampleTime=1e-5  OutDataTypeStr=fixdt(1,64,32)  ICPrevOutput=DiscIntNeverNeededParam  ICPrevScaledInput=DiscIntNeverNeededParam
  Discrete-Time Integrator2 : DiscreteIntegrator  Commented=on  gainval=50  SampleTime=1e-5  OutDataTypeStr=fixdt(1,64,32)  ICPrevOutput=DiscIntNeverNeededParam  ICPrevScaledInput=DiscIntNeverNeededParam
  Discrete-Time Integrator3 : DiscreteIntegrator  gainval=50  SampleTime=1e-5  OutDataTypeStr=fixdt(1,64,32)  ICPrevOutput=DiscIntNeverNeededParam  ICPrevScaledInput=DiscIntNeverNeededParam
  LTI System2 : cstblocks/LTI System  Commented=on  sys=flybackTFD  IC=[]
  Product : Product  OutDataTypeStr=fixdt(1,64,32)
  Product1 : Product  OutDataTypeStr=fixdt(1,64,32)
  Product2 : Product  OutDataTypeStr=fixdt(1,64,32)
  Product3 : Product
  Saturation : Saturate  UpperLimit=255  LowerLimit=0  OutDataTypeStr=fixdt(1,64,32)
  Scope : Scope
  Scope1 : Scope
  Unit Delay : UnitDelay  SampleTime=-1  HasFrameUpgradeWarning=on
  PV : Outport  OutDataTypeStr=fixdt(1,10,0)  SampleTime=0.001  VectorParamsAs1DForOutWhenUnconnected=off
  MV : Outport  Port=2  OutDataTypeStr=fixdt(1,10,0)  SampleTime=0.001  VectorParamsAs1DForOutWhenUnconnected=off
  p_action : Outport  Port=3  OutDataTypeStr=fixdt(1,10,0)  SampleTime=0.001  VectorParamsAs1DForOutWhenUnconnected=off
  i_action : Outport  Port=4  OutDataTypeStr=fixdt(1,10,0)  SampleTime=0.001  VectorParamsAs1DForOutWhenUnconnected=off
  error : Outport  Port=5  OutDataTypeStr=fixdt(1,10,0)  SampleTime=0.001  VectorParamsAs1DForOutWhenUnconnected=off
  wires:
  SP/1 -> Add/1
  Discrete Transfer Fcn1/1 -> Data Type Conversion4/1, Unit Delay/1
  Add/1 -> Data Type Conversion3/1, Product/1, Product1/1
  kp/1 -> Product3/1, Product/2
  Product/1 -> Data Type Conversion1/1, Add1/1
  Discrete-Time Integrator1/1 -> Data Type Conversion5/1, Add1/2
  Unit Delay/1 -> Add/2
  Add1/1 -> Add3/1, Saturation/1
  Product1/1 -> Add2/1
  Add2/1 -> Discrete-Time Integrator1/1
  Add3/1 -> Product2/1
  Product2/1 -> Add2/2
  ti/1 -> Product3/2, Product2/2
  Product3/1 -> Product1/2
  Data Type Conversion3/1 -> error/1  "SP"
  Data Type Conversion1/1 -> p_action/1  "SP"
  Data Type Conversion4/1 -> Scope/1, PV/1  "SP"
  Data Type Conversion2/1 -> Scope1/1, MV/1  "SP"
  Data Type Conversion5/1 -> i_action/1  "SP"
  Saturation/1 -> Discrete-Time Integrator3/1, Data Type Conversion2/1, Add3/2
  Abs/1 -> Discrete Transfer Fcn1/1
  Discrete-Time Integrator3/1 -> Abs/1
